simulink model "simulation"  (R2023a)
settings: Solver=ode4  StartTime=0.0  StopTime=t_duration  FixedStep=dt  RelTol=1e-3
undefined symbols (not defined in the file): gnc, plant, sunPosData
settings Model: Creator=ndelurgio  LastModifiedBy=ndelurgio

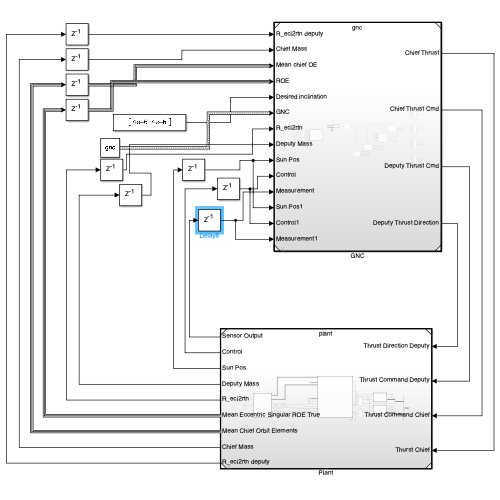
[thumbnail: Simulink's stored preview of the top-level diagram]
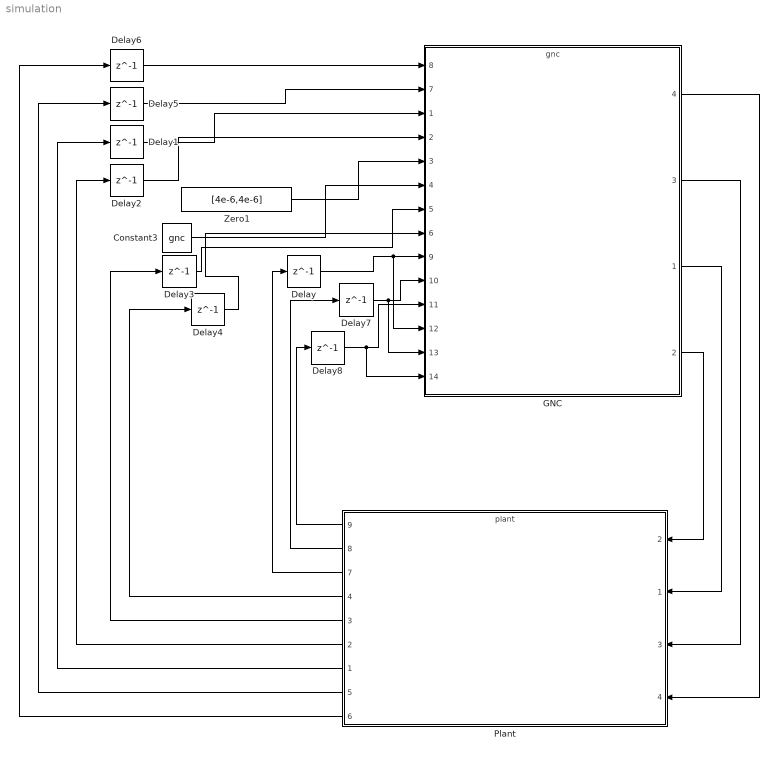
== system simulation ==
  Constant3 : Constant  Value=gnc  OutDataTypeStr=Bus: gncBus
  Delay : Delay  DelayLength=1  InitialCondition=sunPosData(:,1)
  Delay1 : Delay  DelayLength=1  InitialCondition=plant.chief.initialConditions.meanOrbitElements
  Delay2 : Delay  DelayLength=1  InitialCondition=plant.chief.initialConditions.eccentricSingularROE
  Delay3 : Delay  DelayLength=1  InitialCondition=eye(3)
  Delay4 : Delay  DelayLength=1  InitialCondition=plant.deputy.initialConditions.mass_kg
  Delay5 : Delay  DelayLength=1  InitialCondition=plant.chief.initialConditions.mass_kg
  Delay6 : Delay  DelayLength=1  InitialCondition=eye(3)
  Delay7 : Delay  DelayLength=1  InitialCondition=zeros(6,1)
  Delay8 : Delay  DelayLength=1  InitialCondition=gnc.navigation.measurementInit
  GNC : ModelReference  ModelNameDialog=gnc.slx  SimulationMode=Normal  ModelReferenceVersion=1.70
      settings: PortSchema="{\"entries\":[{\"content\":{\"sides\":[{\"content\":{\"connectorIds\":[\"In8\",\"In7\",\"In1\",\"In2\",\"In3\",\"In4\",\"In5\",\"In6\",\"In9\",\"In10\",\"In11\",\"In12\",\"In13\",\"In14\"]},\"type\":\"ConnectorPlacement.EquallySpacedRectSide\",\"uuid\":\"7593418b-06da-4437-822b-6ce939d5abc1\"},{\"content\":{\"connectorIds\":[\"Out4\",\"Out3\",\"Out1\",\"Out2\"],\"side\":\"RIGHT\"},\"type\":\"ConnectorPlacement.EquallySpacedRectSide\",\"uuid\":\"90307b6c-4c19-4df5-a59b-edb1e3ede9d3\"},{\"content\":{\"side\":\"TOP\"},\"type\":\"ConnectorPlacement.EquallySpacedRectSide\",\"uuid\":\"59305b16-fd05-4946-aed7-57e576ca8484\"}]},\"type\":\"ConnectorPlacement.EquallySpacedConnector\",\"uuid\":\"65f9b4f5-3c44-44c1-99bd-5ae1f7debbe5\"}],\"packageUris\":[\"http://schema.mathworks.com/mf0/Connector/R2020b\"],\"version\":\"1.0\"}"
  Plant : ModelReference  ModelNameDialog=plant.slx  SimulationMode=Normal  ModelReferenceVersion=1.52
      settings: PortSchema="{\"entries\":[{\"content\":{\"sides\":[{\"content\":{\"connectorIds\":[\"In2\",\"In1\",\"In3\",\"In4\"]},\"type\":\"ConnectorPlacement.EquallySpacedRectSide\",\"uuid\":\"f73cb6fc-3242-4a7e-989f-6a11f9cf0691\"},{\"content\":{\"connectorIds\":[\"Out9\",\"Out8\",\"Out7\",\"Out4\",\"Out3\",\"Out2\",\"Out1\",\"Out5\",\"Out6\"],\"side\":\"RIGHT\"},\"type\":\"ConnectorPlacement.EquallySpacedRectSide\",\"uuid\":\"4e8b4bfa-81a4-4dd6-b255-9cd934ba946d\"},{\"content\":{\"side\":\"TOP\"},\"type\":\"ConnectorPlacement.EquallySpacedRectSide\",\"uuid\":\"fbcf9ade-d9d9-43d2-bc74-e365e7bd56cd\"}]},\"type\":\"ConnectorPlacement.EquallySpacedConnector\",\"uuid\":\"ad9fbc43-81a6-43cd-b12b-520ff2a805d7\"}],\"packageUris\":[\"http://schema.mathworks.com/mf0/Connector/R2020b\"],\"version\":\"1.0\"}"
  Zero1 : Constant  Value=[4e-6,4e-6]  OutDataTypeStr=Inherit: Inherit via back propagation
  wires:
  Plant/1 -> Delay1/1
  Plant/2 -> Delay2/1
  Plant/3 -> Delay3/1
  Plant/4 -> Delay4/1
  GNC/1 -> Plant/1
  GNC/2 -> Plant/2
  Zero1/1 -> GNC/3
  Constant3/1 -> GNC/4
  Delay1/1 -> GNC/1
  Delay2/1 -> GNC/2
  Delay3/1 -> GNC/5
  Delay4/1 -> GNC/6
  GNC/4 -> Plant/4
  GNC/3 -> Plant/3
  Plant/5 -> Delay5/1
  Delay5/1 -> GNC/7
  Plant/6 -> Delay6/1
  Delay6/1 -> GNC/8
  Plant/7 -> Delay/1
  Plant/8 -> Delay7/1
  Plant/9 -> Delay8/1
  Delay/1 -> GNC/12, GNC/9
  Delay7/1 -> GNC/13, GNC/10
  Delay8/1 -> GNC/14, GNC/11
